simulink model "hinfinity"  (R2021a)
settings: Solver=VariableStepAuto  StartTime=0.0  StopTime=10  RelTol=1e-3  EnableMultiTasking=on
values from neighbouring files (symbols this model uses):
  A = [ 0 1 0 0 0 0 0 0 ... (first row only)    [robust_control.m]
  b = 3.13*10^-5    (= 3.13e-05)    [robust_control.m]
  B = [0 0 0 0 ... (first row only)    [robust_control.m]
  BW = [0 0 0 0 1 0 0 ... (first row only)    [robust_control.m]
  C = [ 1 0 0 0 0 0 0 0 ... (first row only)    [robust_control.m]
  d = 7.5*10^-7    (= 7.5e-07)    [robust_control.m]
  D = [0 0 0 0 ... (first row only)    [robust_control.m]
  DW = [0 0 0 0 0 0 0 ... (first row only)    [robust_control.m]
  l = 0.23    [robust_control.m]
  om = 200^2    (= 40000)    [robust_control.m]
  om2 = 100^2    (= 10000)    [robust_control.m]
undefined symbols (not defined in the file or in its folder): K
libraries: pid_lib x4, cstblocks x3, simulink x2
settings Model: Creator=engrh  LastModifiedBy=itcef
settings SolverCC: AlgebraicLoopSolver=TrustRegion
settings DataIOCC: ReturnWorkspaceOutputs=off
settings OptimizationCC: DefaultParameterBehavior=Inlined  BufferReuse=off  LifeSpan=inf
settings DebuggingCC: InitInArrayFormatMsg=none  SFUnexpectedBacktrackingDiag=warning  SFNoUnconditionalDefaultTransitionDiag=warning  SFMachineParentedDataDiag=warning  ArithmeticOperatorsInVariantConditions=warning
settings SFSimCC: SimUseLocalCustomCode=off  CustomCodeUndefinedFunction=UseInterfaceOnly
settings RTWCC: RTWUseLocalCustomCode=off
settings CodeAppCC: StateflowObjectComments=on
settings GRTTargetCC: TargetLangStandard=C89/C90 (ANSI)
settings ConfigComp: CovMetricSettings=dw  CovSaveCumulativeToWorkspaceVar=on  CovSaveSingleToWorkspaceVar=on  CovExternalEMLEnable=off

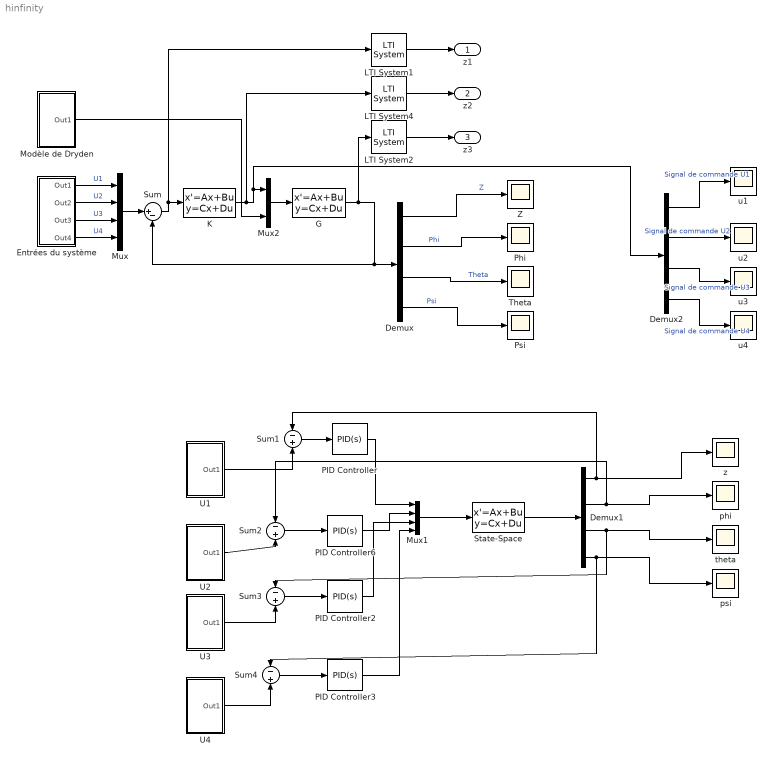
== system hinfinity ==
  Demux : Demux
  Demux1 : Demux
  Demux2 : Demux
  Entrées du système : Subsystem
  G : StateSpace  A=A  B=BW  C=C  D=DW  InitialCondition=0
  K : StateSpace  A=K.A  B=K.B  C=K.C  D=K.D  InitialCondition=0
  LTI System1 : cstblocks/LTI System  sys=W1  IC=[]
  LTI System2 : cstblocks/LTI System  sys=W3  IC=[]
  LTI System4 : cstblocks/LTI System  sys=W2  IC=[]
  Modèle de Dryden : Subsystem
  Mux : Mux
  Mux1 : Mux
  Mux2 : Mux  Inputs=2
  PID Controller : pid_lib/PID Controller  Controller=PID  Form=Parallel  TimeDomain=Continuous-time  UseExternalTs=off  SampleTime=-1  IntegratorMethod=Forward Euler  FilterMethod=Forward Euler  ControllerParametersSource=internal  P=5.58109752030264  I=1.80241201307742  D=4.10370707631122  UseFilter=on  N=16.3080880799928  TunerSelectOption=Transfer Function Based (PID Tuner App)  InitialConditionSource=internal  InitialConditionForIntegrator=0  InitialConditionForFilter=0  DifferentiatorICPrevScaledInput=0  ExternalReset=none  TrackingMode=off  Kt=1  LimitOutput=off  SatLimitsSource=internal  UpperSaturationLimit=inf  LowerSaturationLimit=-inf  LinearizeAsGain=on  AntiWindupMode=none  Kb=1  POutMin=[]  POutMax=[]  IOutMin=[]  IOutMax=[]  DOutMin=[]  DOutMax=[]  NOutMin=[]  NOutMax=[]  SumOutMin=[]  SumOutMax=[]  SaturationOutMin=[]  SaturationOutMax=[]  PParamMin=[]  PParamMax=[]  IParamMin=[]  IParamMax=[]  DParamMin=[]  DParamMax=[]  NParamMin=[]  NParamMax=[]  KbParamMin=[]  KbParamMax=[]  KtParamMin=[]  KtParamMax=[]  KbOutMin=[]  KbOutMax=[]  KtOutMin=[]  KtOutMax=[]  IntegratorOutMin=[]  IntegratorOutMax=[]  FilterOutMin=[]  FilterOutMax=[]  SumI1OutMin=[]  SumI1OutMax=[]  SumI2OutMin=[]  SumI2OutMax=[]  SumI3OutMin=[]  SumI3OutMax=[]  SumI4OutMin=[]  SumI4OutMax=[]  SumDOutMin=[]  SumDOutMax=[]  DifferentiatorOutMin=[]  DifferentiatorOutMax=[]  FilterDiffOutCoefMin=[]  FilterDiffOutCoefMax=[]  ReciprocalOutMin=[]  ReciprocalOutMax=[]  SumDenOutMin=[]  SumDenOutMax=[]  SumNumOutMin=[]  SumNumOutMax=[]  DivideOutMin=[]  DivideOutMax=[]  UdiffTsProdOutMin=[]  UdiffTsProdOutMax=[]  NTsProdOutMin=[]  NTsProdOutMax=[]  UintegralTsProdOutMin=[]  UintegralTsProdOutMax=[]  UngainTsProdOutMin=[]  UngainTsProdOutMax=[]  IntegratorContinuousStateAttributes=''  IntegratorStateMustResolveToSignalObject=off  IntegratorRTWStateStorageClass=Auto  FilterContinuousStateAttributes=''  FilterStateMustResolveToSignalObject=off  FilterRTWStateStorageClass=Auto  ParallelPVariant=InternalParameters  IdealPVariant=Disabled  IVariant=InternalParameters  DVariant=InternalParameters  IntegratorVariant=Continuous  SatVariant=Disabled  AWVariant=Passthrough  PCopyVariant=Disabled  TRVariant=Disabled  FdbkBlocksVariant=Forward  IdealPFdbkVariant=Disabled  SatFdbkVariant=Disabled  DerivativeFilterVariant=ContFilter  NVariant=InternalParameters  NCopyVariant=Disabled  FilterICVariant=InternalICsFilter  IntegratorICVariant=InternalICs  ExternalResetVariant=Disabled  TRSumVariant=Passthrough  SumFdbkVariant=Disabled  SumVariant=Sum_PID  TsampFilterVariant=InternalTs  TsampNgainVariant=Passthrough  TsampIntegralVariant=Passthrough  ExternalSaturationOutDataTypeStr=Inherit: Same as second input
  PID Controller2 : pid_lib/PID Controller  Controller=PID  Form=Parallel  TimeDomain=Continuous-time  UseExternalTs=off  SampleTime=-1  IntegratorMethod=Forward Euler  FilterMethod=Forward Euler  ControllerParametersSource=internal  P=0.000723812316024167  I=2.123608634526e-05  D=0.00451289281425092  UseFilter=on  N=3.44122258847421  TunerSelectOption=Transfer Function Based (PID Tuner App)  InitialConditionSource=internal  InitialConditionForIntegrator=0  InitialConditionForFilter=0  DifferentiatorICPrevScaledInput=0  ExternalReset=none  TrackingMode=off  Kt=1  LimitOutput=off  SatLimitsSource=internal  UpperSaturationLimit=inf  LowerSaturationLimit=-inf  LinearizeAsGain=on  AntiWindupMode=none  Kb=1  POutMin=[]  POutMax=[]  IOutMin=[]  IOutMax=[]  DOutMin=[]  DOutMax=[]  NOutMin=[]  NOutMax=[]  SumOutMin=[]  SumOutMax=[]  SaturationOutMin=[]  SaturationOutMax=[]  PParamMin=[]  PParamMax=[]  IParamMin=[]  IParamMax=[]  DParamMin=[]  DParamMax=[]  NParamMin=[]  NParamMax=[]  KbParamMin=[]  KbParamMax=[]  KtParamMin=[]  KtParamMax=[]  KbOutMin=[]  KbOutMax=[]  KtOutMin=[]  KtOutMax=[]  IntegratorOutMin=[]  IntegratorOutMax=[]  FilterOutMin=[]  FilterOutMax=[]  SumI1OutMin=[]  SumI1OutMax=[]  SumI2OutMin=[]  SumI2OutMax=[]  SumI3OutMin=[]  SumI3OutMax=[]  SumI4OutMin=[]  SumI4OutMax=[]  SumDOutMin=[]  SumDOutMax=[]  DifferentiatorOutMin=[]  DifferentiatorOutMax=[]  FilterDiffOutCoefMin=[]  FilterDiffOutCoefMax=[]  ReciprocalOutMin=[]  ReciprocalOutMax=[]  SumDenOutMin=[]  SumDenOutMax=[]  SumNumOutMin=[]  SumNumOutMax=[]  DivideOutMin=[]  DivideOutMax=[]  UdiffTsProdOutMin=[]  UdiffTsProdOutMax=[]  NTsProdOutMin=[]  NTsProdOutMax=[]  UintegralTsProdOutMin=[]  UintegralTsProdOutMax=[]  UngainTsProdOutMin=[]  UngainTsProdOutMax=[]  IntegratorContinuousStateAttributes=''  IntegratorStateMustResolveToSignalObject=off  IntegratorRTWStateStorageClass=Auto  FilterContinuousStateAttributes=''  FilterStateMustResolveToSignalObject=off  FilterRTWStateStorageClass=Auto  ParallelPVariant=InternalParameters  IdealPVariant=Disabled  IVariant=InternalParameters  DVariant=InternalParameters  IntegratorVariant=Continuous  SatVariant=Disabled  AWVariant=Passthrough  PCopyVariant=Disabled  TRVariant=Disabled  FdbkBlocksVariant=Forward  IdealPFdbkVariant=Disabled  SatFdbkVariant=Disabled  DerivativeFilterVariant=ContFilter  NVariant=InternalParameters  NCopyVariant=Disabled  FilterICVariant=InternalICsFilter  IntegratorICVariant=InternalICs  ExternalResetVariant=Disabled  TRSumVariant=Passthrough  SumFdbkVariant=Disabled  SumVariant=Sum_PID  TsampFilterVariant=InternalTs  TsampNgainVariant=Passthrough  TsampIntegralVariant=Passthrough  ExternalSaturationOutDataTypeStr=Inherit: Same as second input
  PID Controller3 : pid_lib/PID Controller  Controller=PID  Form=Parallel  TimeDomain=Continuous-time  UseExternalTs=off  SampleTime=-1  IntegratorMethod=Forward Euler  FilterMethod=Forward Euler  ControllerParametersSource=internal  P=0.00198841970129611  I=7.34440421903456e-05  D=0.00984775210391055  UseFilter=on  N=4.33224256427029  TunerSelectOption=Transfer Function Based (PID Tuner App)  InitialConditionSource=internal  InitialConditionForIntegrator=0  InitialConditionForFilter=0  DifferentiatorICPrevScaledInput=0  ExternalReset=none  TrackingMode=off  Kt=1  LimitOutput=off  SatLimitsSource=internal  UpperSaturationLimit=inf  LowerSaturationLimit=-inf  LinearizeAsGain=on  AntiWindupMode=none  Kb=1  POutMin=[]  POutMax=[]  IOutMin=[]  IOutMax=[]  DOutMin=[]  DOutMax=[]  NOutMin=[]  NOutMax=[]  SumOutMin=[]  SumOutMax=[]  SaturationOutMin=[]  SaturationOutMax=[]  PParamMin=[]  PParamMax=[]  IParamMin=[]  IParamMax=[]  DParamMin=[]  DParamMax=[]  NParamMin=[]  NParamMax=[]  KbParamMin=[]  KbParamMax=[]  KtParamMin=[]  KtParamMax=[]  KbOutMin=[]  KbOutMax=[]  KtOutMin=[]  KtOutMax=[]  IntegratorOutMin=[]  IntegratorOutMax=[]  FilterOutMin=[]  FilterOutMax=[]  SumI1OutMin=[]  SumI1OutMax=[]  SumI2OutMin=[]  SumI2OutMax=[]  SumI3OutMin=[]  SumI3OutMax=[]  SumI4OutMin=[]  SumI4OutMax=[]  SumDOutMin=[]  SumDOutMax=[]  DifferentiatorOutMin=[]  DifferentiatorOutMax=[]  FilterDiffOutCoefMin=[]  FilterDiffOutCoefMax=[]  ReciprocalOutMin=[]  ReciprocalOutMax=[]  SumDenOutMin=[]  SumDenOutMax=[]  SumNumOutMin=[]  SumNumOutMax=[]  DivideOutMin=[]  DivideOutMax=[]  UdiffTsProdOutMin=[]  UdiffTsProdOutMax=[]  NTsProdOutMin=[]  NTsProdOutMax=[]  UintegralTsProdOutMin=[]  UintegralTsProdOutMax=[]  UngainTsProdOutMin=[]  UngainTsProdOutMax=[]  IntegratorContinuousStateAttributes=''  IntegratorStateMustResolveToSignalObject=off  IntegratorRTWStateStorageClass=Auto  FilterContinuousStateAttributes=''  FilterStateMustResolveToSignalObject=off  FilterRTWStateStorageClass=Auto  ParallelPVariant=InternalParameters  IdealPVariant=Disabled  IVariant=InternalParameters  DVariant=InternalParameters  IntegratorVariant=Continuous  SatVariant=Disabled  AWVariant=Passthrough  PCopyVariant=Disabled  TRVariant=Disabled  FdbkBlocksVariant=Forward  IdealPFdbkVariant=Disabled  SatFdbkVariant=Disabled  DerivativeFilterVariant=ContFilter  NVariant=InternalParameters  NCopyVariant=Disabled  FilterICVariant=InternalICsFilter  IntegratorICVariant=InternalICs  ExternalResetVariant=Disabled  TRSumVariant=Passthrough  SumFdbkVariant=Disabled  SumVariant=Sum_PID  TsampFilterVariant=InternalTs  TsampNgainVariant=Passthrough  TsampIntegralVariant=Passthrough  ExternalSaturationOutDataTypeStr=Inherit: Same as second input
  PID Controller6 : pid_lib/PID Controller  Controller=PID  Form=Parallel  TimeDomain=Continuous-time  UseExternalTs=off  SampleTime=-1  IntegratorMethod=Forward Euler  FilterMethod=Forward Euler  ControllerParametersSource=internal  P=0.00119316717565162  I=5.1954532977315e-05  D=0.00667135540634302  UseFilter=on  N=3.32594307811915  TunerSelectOption=Transfer Function Based (PID Tuner App)  InitialConditionSource=internal  InitialConditionForIntegrator=0  InitialConditionForFilter=0  DifferentiatorICPrevScaledInput=0  ExternalReset=none  TrackingMode=off  Kt=1  LimitOutput=off  SatLimitsSource=internal  UpperSaturationLimit=inf  LowerSaturationLimit=-inf  LinearizeAsGain=on  AntiWindupMode=none  Kb=1  POutMin=[]  POutMax=[]  IOutMin=[]  IOutMax=[]  DOutMin=[]  DOutMax=[]  NOutMin=[]  NOutMax=[]  SumOutMin=[]  SumOutMax=[]  SaturationOutMin=[]  SaturationOutMax=[]  PParamMin=[]  PParamMax=[]  IParamMin=[]  IParamMax=[]  DParamMin=[]  DParamMax=[]  NParamMin=[]  NParamMax=[]  KbParamMin=[]  KbParamMax=[]  KtParamMin=[]  KtParamMax=[]  KbOutMin=[]  KbOutMax=[]  KtOutMin=[]  KtOutMax=[]  IntegratorOutMin=[]  IntegratorOutMax=[]  FilterOutMin=[]  FilterOutMax=[]  SumI1OutMin=[]  SumI1OutMax=[]  SumI2OutMin=[]  SumI2OutMax=[]  SumI3OutMin=[]  SumI3OutMax=[]  SumI4OutMin=[]  SumI4OutMax=[]  SumDOutMin=[]  SumDOutMax=[]  DifferentiatorOutMin=[]  DifferentiatorOutMax=[]  FilterDiffOutCoefMin=[]  FilterDiffOutCoefMax=[]  ReciprocalOutMin=[]  ReciprocalOutMax=[]  SumDenOutMin=[]  SumDenOutMax=[]  SumNumOutMin=[]  SumNumOutMax=[]  DivideOutMin=[]  DivideOutMax=[]  UdiffTsProdOutMin=[]  UdiffTsProdOutMax=[]  NTsProdOutMin=[]  NTsProdOutMax=[]  UintegralTsProdOutMin=[]  UintegralTsProdOutMax=[]  UngainTsProdOutMin=[]  UngainTsProdOutMax=[]  IntegratorContinuousStateAttributes=''  IntegratorStateMustResolveToSignalObject=off  IntegratorRTWStateStorageClass=Auto  FilterContinuousStateAttributes=''  FilterStateMustResolveToSignalObject=off  FilterRTWStateStorageClass=Auto  ParallelPVariant=InternalParameters  IdealPVariant=Disabled  IVariant=InternalParameters  DVariant=InternalParameters  IntegratorVariant=Continuous  SatVariant=Disabled  AWVariant=Passthrough  PCopyVariant=Disabled  TRVariant=Disabled  FdbkBlocksVariant=Forward  IdealPFdbkVariant=Disabled  SatFdbkVariant=Disabled  DerivativeFilterVariant=ContFilter  NVariant=InternalParameters  NCopyVariant=Disabled  FilterICVariant=InternalICsFilter  IntegratorICVariant=InternalICs  ExternalResetVariant=Disabled  TRSumVariant=Passthrough  SumFdbkVariant=Disabled  SumVariant=Sum_PID  TsampFilterVariant=InternalTs  TsampNgainVariant=Passthrough  TsampIntegralVariant=Passthrough  ExternalSaturationOutDataTypeStr=Inherit: Same as second input
  Phi : Scope
  Psi : Scope
  State-Space : StateSpace  A=A  B=B  C=C  D=D  InitialCondition=0
  Sum : Sum  Inputs=|+-
  Sum{1..4} (4 alike) : Sum  Inputs=-+
  Theta : Scope
  U1 : Subsystem
  "U2 " : Subsystem
  U3 : Subsystem
  U4 : Subsystem
  Z : Scope
  phi : Scope
  psi : Scope
  theta : Scope
  u{1..4} (4 alike) : Scope
  z : Scope
  z1 : Outport
  z2 : Outport  Port=2
  z3 : Outport  Port=3
  wires:
  Mux/1 -> Sum/1
  G/1 -> Sum/2, Demux/1, LTI System2/1
  Demux/2 -> Phi/1  "Phi"
  Demux/3 -> Theta/1  "Theta"
  Demux/4 -> Psi/1  "Psi"
  Entrées du système/1(Out1) -> Mux/1  "U1"
  Entrées du système/2(Out2) -> Mux/2  "U2"
  Entrées du système/3(Out3) -> Mux/3  "U3"
  Entrées du système/4(Out4) -> Mux/4  "U4"
  Demux1/4 -> Sum4/1, psi/1
  State-Space/1 -> Demux1/1
  U1/1(Out1) -> Sum1/2
  Sum4/1 -> PID Controller3/1
  Demux1/1 -> z/1, Sum1/1
  Sum1/1 -> PID Controller/1
  Sum2/1 -> PID Controller6/1
  U4/1(Out1) -> Sum4/2
  U3/1(Out1) -> Sum3/2
  Demux1/3 -> theta/1, Sum3/1
  Demux1/2 -> phi/1, Sum2/1
  Sum3/1 -> PID Controller2/1
  "U2 "/1(Out1) -> Sum2/2
  Demux/1 -> Z/1  "Z"
  Sum/1 -> LTI System1/1, K/1
  Mux1/1 -> State-Space/1
  PID Controller/1 -> Mux1/1
  PID Controller6/1 -> Mux1/2
  PID Controller2/1 -> Mux1/3
  PID Controller3/1 -> Mux1/4
  LTI System1/1 -> z1/1
  LTI System4/1 -> z2/1
  LTI System2/1 -> z3/1
  Mux2/1 -> G/1
  K/1 -> LTI System4/1, Demux2/1, Mux2/1
  Demux2/2 -> u2/1  "Signal de commande U2"
  Demux2/3 -> u3/1  "Signal de commande U3"
  Demux2/4 -> u4/1  "Signal de commande U4"
  Demux2/1 -> u1/1  "Signal de commande U1"
  Modèle de Dryden/1(Out1) -> Mux2/2

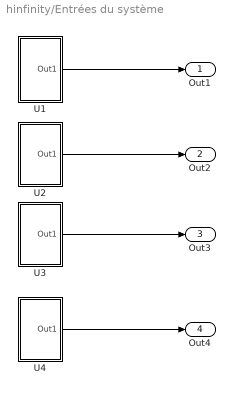
== system hinfinity/Entrées du système ==
  U1 : Subsystem
  "U2 " : Subsystem
  U3 : Subsystem
  U4 : Subsystem
  Out1 : Outport
  Out2 : Outport  Port=2
  Out3 : Outport  Port=3
  Out4 : Outport  Port=4
  wires:
  U1/1(Out1) -> Out1/1
  U4/1(Out1) -> Out4/1
  U3/1(Out1) -> Out3/1
  "U2 "/1(Out1) -> Out2/1

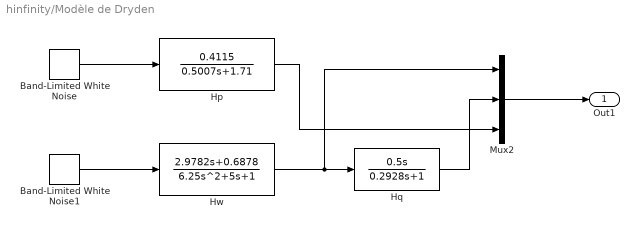
== system hinfinity/Modèle de Dryden ==
  Band-Limited White Noise : simulink/Sources/Band-Limited White Noise  Cov=[0.01]  Ts=0.1  seed=[2508741]
  Band-Limited White Noise1 : simulink/Sources/Band-Limited White Noise  Cov=[0.01]  Ts=0.1  seed=[2502241]
  Hp : TransferFcn  Numerator=[0.4115]  Denominator=[ 0.5007 1.71]
  Hq : TransferFcn  Numerator=[0.5 0]  Denominator=[0.2928 1]
  Hw : TransferFcn  Numerator=[2.9782 0.6878]  Denominator=[6.25 5 1]
  Mux2 : Mux  Inputs=3
  Out1 : Outport
  wires:
  Hw/1 -> Mux2/1, Hq/1
  Mux2/1 -> Out1/1
  Band-Limited White Noise1/1 -> Hw/1
  Hp/1 -> Mux2/3
  Hq/1 -> Mux2/2
  Band-Limited White Noise/1 -> Hp/1

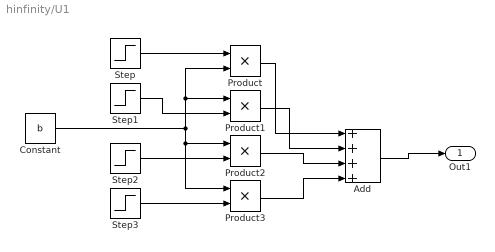
== system hinfinity/U1 ==
  Add : Sum  Inputs=++++
  Constant : Constant  Value=b
  Product{,1..3} (4 alike) : Product
  Step{,1..3} (4 alike) : Step  Time=0  After=om  SampleTime=0
  Out1 : Outport
  wires:
  Constant/1 -> Product1/1, Product/2, Product2/1, Product3/1
  Product1/1 -> Add/2
  Step3/1 -> Product3/2
  Step2/1 -> Product2/2
  Product3/1 -> Add/4
  Step1/1 -> Product1/2
  Step/1 -> Product/1
  Product/1 -> Add/1
  Product2/1 -> Add/3
  Add/1 -> Out1/1

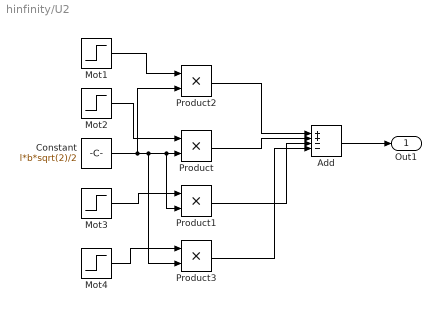
== system hinfinity/U2  ==
  Add : Sum  Inputs=++--
  Constant : Constant  Value=l*b*sqrt(2)/2
  Mot1 : Step  Time=2  After=om  SampleTime=0
  Mot2 : Step  Time=2  After=om  SampleTime=0
  Mot3 : Step  Time=2  After=om2  SampleTime=0
  Mot4 : Step  Time=2  After=om2  SampleTime=0
  Product{,1..3} (4 alike) : Product
  Out1 : Outport
  wires:
  Mot4/1 -> Product3/1
  Constant/1 -> Product2/2, Product3/2, Product1/2, Product/2
  Mot3/1 -> Product1/1
  Mot1/1 -> Product2/1
  Product1/1 -> Add/3
  Product/1 -> Add/2
  Product3/1 -> Add/4
  Mot2/1 -> Product/1
  Product2/1 -> Add/1
  Add/1 -> Out1/1

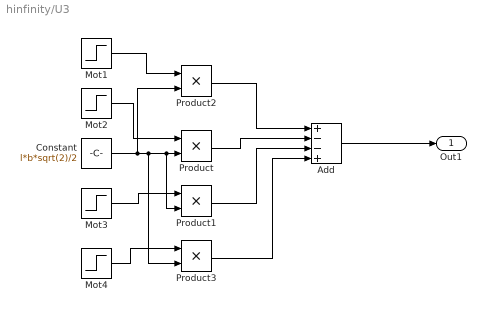
== system hinfinity/U3 ==
  Add : Sum  Inputs=+--+
  Constant : Constant  Value=l*b*sqrt(2)/2
  Mot1 : Step  Time=2  After=om  SampleTime=0
  Mot2 : Step  Time=2  After=om2  SampleTime=0
  Mot3 : Step  Time=2  After=om2  SampleTime=0
  Mot4 : Step  Time=2  After=om  SampleTime=0
  Product{,1..3} (4 alike) : Product
  Out1 : Outport
  wires:
  Mot4/1 -> Product3/1
  Product1/1 -> Add/3
  Mot1/1 -> Product2/1
  Product2/1 -> Add/1
  Add/1 -> Out1/1
  Mot3/1 -> Product1/1
  Constant/1 -> Product2/2, Product3/2, Product1/2, Product/2
  Product/1 -> Add/2
  Mot2/1 -> Product/1
  Product3/1 -> Add/4

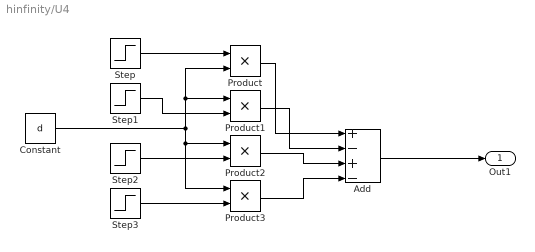
== system hinfinity/U4 ==
  Add : Sum  Inputs=+-+-
  Constant : Constant  Value=d
  Product{,1..3} (4 alike) : Product
  Step : Step  Time=2  After=om  SampleTime=0
  Step1 : Step  Time=2  After=om2  SampleTime=0
  Step2 : Step  Time=2  After=om  SampleTime=0
  Step3 : Step  Time=2  After=om2  SampleTime=0
  Out1 : Outport
  wires:
  Step1/1 -> Product1/2
  Step2/1 -> Product2/2
  Product1/1 -> Add/2
  Product2/1 -> Add/3
  Product3/1 -> Add/4
  Product/1 -> Add/1
  Constant/1 -> Product1/1, Product/2, Product2/1, Product3/1
  Step3/1 -> Product3/2
  Step/1 -> Product/1
  Add/1 -> Out1/1

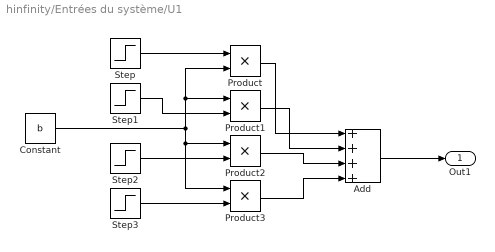
== system hinfinity/Entrées du système/U1 ==
  Add : Sum  Inputs=++++
  Constant : Constant  Value=b
  Product{,1..3} (4 alike) : Product
  Step{,1..3} (4 alike) : Step  Time=0  After=om  SampleTime=0
  Out1 : Outport
  wires:
  Constant/1 -> Product1/1, Product/2, Product2/1, Product3/1
  Product1/1 -> Add/2
  Step3/1 -> Product3/2
  Step2/1 -> Product2/2
  Product3/1 -> Add/4
  Step1/1 -> Product1/2
  Step/1 -> Product/1
  Product/1 -> Add/1
  Product2/1 -> Add/3
  Add/1 -> Out1/1

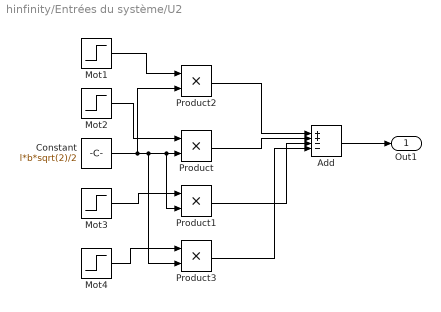
== system hinfinity/Entrées du système/U2  ==
  Add : Sum  Inputs=++--
  Constant : Constant  Value=l*b*sqrt(2)/2
  Mot1 : Step  Time=2  After=om  SampleTime=0
  Mot2 : Step  Time=2  After=om  SampleTime=0
  Mot3 : Step  Time=2  After=om2  SampleTime=0
  Mot4 : Step  Time=2  After=om2  SampleTime=0
  Product{,1..3} (4 alike) : Product
  Out1 : Outport
  wires:
  Mot4/1 -> Product3/1
  Constant/1 -> Product2/2, Product3/2, Product1/2, Product/2
  Mot3/1 -> Product1/1
  Mot1/1 -> Product2/1
  Product1/1 -> Add/3
  Product/1 -> Add/2
  Product3/1 -> Add/4
  Mot2/1 -> Product/1
  Product2/1 -> Add/1
  Add/1 -> Out1/1

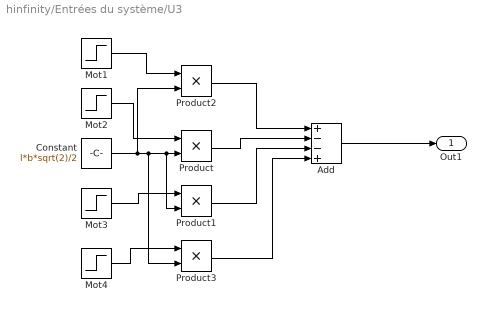
== system hinfinity/Entrées du système/U3 ==
  Add : Sum  Inputs=+--+
  Constant : Constant  Value=l*b*sqrt(2)/2
  Mot1 : Step  Time=4  After=om  SampleTime=0
  Mot2 : Step  Time=4  After=om2  SampleTime=0
  Mot3 : Step  Time=4  After=om2  SampleTime=0
  Mot4 : Step  Time=4  After=om  SampleTime=0
  Product{,1..3} (4 alike) : Product
  Out1 : Outport
  wires:
  Mot4/1 -> Product3/1
  Product1/1 -> Add/3
  Mot1/1 -> Product2/1
  Product2/1 -> Add/1
  Add/1 -> Out1/1
  Mot3/1 -> Product1/1
  Constant/1 -> Product2/2, Product3/2, Product1/2, Product/2
  Product/1 -> Add/2
  Mot2/1 -> Product/1
  Product3/1 -> Add/4

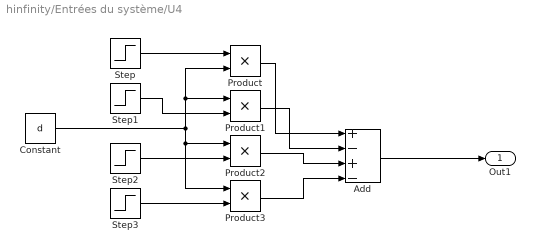
== system hinfinity/Entrées du système/U4 ==
  Add : Sum  Inputs=+-+-
  Constant : Constant  Value=d
  Product{,1..3} (4 alike) : Product
  Step : Step  Time=6  After=om  SampleTime=0
  Step1 : Step  Time=6  After=om2  SampleTime=0
  Step2 : Step  Time=6  After=om  SampleTime=0
  Step3 : Step  Time=6  After=om2  SampleTime=0
  Out1 : Outport
  wires:
  Step1/1 -> Product1/2
  Step2/1 -> Product2/2
  Product1/1 -> Add/2
  Product2/1 -> Add/3
  Product3/1 -> Add/4
  Product/1 -> Add/1
  Constant/1 -> Product1/1, Product/2, Product2/1, Product3/1
  Step3/1 -> Product3/2
  Step/1 -> Product/1
  Add/1 -> Out1/1
